simulink model "parmest"  (Simulink 6.0)
settings: Solver=ode45  SolverMode=SingleTasking  StartTime=0.0  StopTime=10000  RelTol=1e-3  AbsTol=1e-6
settings Model: Creator=The MathWorks Inc.  LastModifiedBy=batserve  ExtModeTrigMode=oneshot  ExtModeAutoUpdateStatusClock=off
settings DataIOCC: ExternalInput=[]  InitialState=[]  LimitDataPoints=off  SaveOutput=off  SaveTime=off
settings OptimizationCC: BooleanDataType=off
settings DebuggingCC: CheckExecutionContextPreStartOutputMsg=on  CheckExecutionContextRuntimeOutputMsg=on  SolverPrmCheckMsg=none
settings HardwareCC: TargetUnknown=on

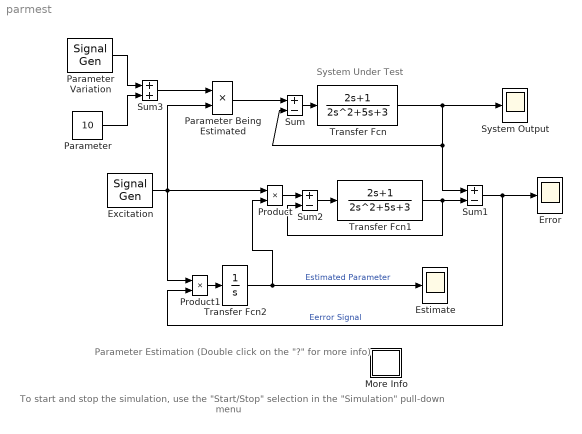
== system parmest ==
  note: To start and stop the simulation, use the "Start/Stop"
      | selection in the "Simulation" pull-down menu
  note: Parameter Estimation
      | (Double click on the "?" for more info)
  note: System Under Test
  Error : Scope
      settings: TickLabels=on  TimeRange=150  YMin=-3  YMax=3  DataFormat=Array
  Estimate : Scope
      settings: TickLabels=on  TimeRange=150  YMin=6  YMax=14  DataFormat=Array
  Excitation : SignalGenerator  WaveForm=sawtooth  Amplitude=1.940000  Frequency=2.000000  Units=rad/sec
  More Info : Subsystem  PropExecContextAcrossSSBoundary=on
      mask Display: disp('?')
  Parameter : Constant  Value=10
  Parameter Being Estimated : Product  SaturateOnIntegerOverflow=on  RndMeth=Zero  InputSameDT=on
  Parameter Variation : SignalGenerator  WaveForm=square  Amplitude=4.000000  Frequency=0.100000  Units=rad/sec
  Product : Product  SaturateOnIntegerOverflow=on  RndMeth=Zero  InputSameDT=on
  Product1 : Product  SaturateOnIntegerOverflow=on  RndMeth=Zero  InputSameDT=on
  Sum : Sum  Inputs=+-  SaturateOnIntegerOverflow=on  InputSameDT=on
  Sum1 : Sum  Inputs=+-  SaturateOnIntegerOverflow=on  InputSameDT=on
  Sum2 : Sum  Inputs=+-  SaturateOnIntegerOverflow=on  InputSameDT=on
  Sum3 : Sum  SaturateOnIntegerOverflow=on  InputSameDT=on
  System Output : Scope
      settings: TickLabels=on  TimeRange=150  YMin=-7.5  YMax=7.5  DataFormat=Array
  Transfer Fcn : TransferFcn  Numerator=[2,1]  Denominator=[2,5,3]
  Transfer Fcn1 : TransferFcn  Numerator=[2,1]  Denominator=[2,5,3]
  Transfer Fcn2 : TransferFcn  Denominator=[1,0]
  wires:
  Product/1 -> Sum2/1
  Sum2/1 -> Transfer Fcn1/1
  Transfer Fcn1/1 -> Sum1/2, Sum2/2
  Product1/1 -> Transfer Fcn2/1
  Transfer Fcn2/1 -> Estimate/1, Product/2  "Estimated Parameter"
  Sum1/1 -> Error/1, Product1/2  "Eerror Signal"
  Parameter Being Estimated/1 -> Sum/1
  Sum/1 -> Transfer Fcn/1
  Transfer Fcn/1 -> System Output/1, Sum1/1, Sum/2
  Excitation/1 -> Parameter Being Estimated/2, Product1/1, Product/1
  Parameter Variation/1 -> Sum3/1
  Parameter/1 -> Sum3/2
  Sum3/1 -> Parameter Being Estimated/1

== system parmest/More Info ==
  note: Watch the system estimate and error respond as the
      | gain parameter changes during the simulation.
  note: This system estimates a single scalar parameter.
      | Open the scopes and run the simulation.
  note: The changing value of the gain applied in the
      | Product block "Parameter being estimated" is
      | the quantity being estimated.
